simulink subsystem "Hall_Sensor_Reader"  (R2024b)
settings: Solver=VariableStepAuto  StartTime=0.0  StopTime=10.0  RelTol=1e-3
settings Model: Creator=luigi  LastModifiedBy=luigi

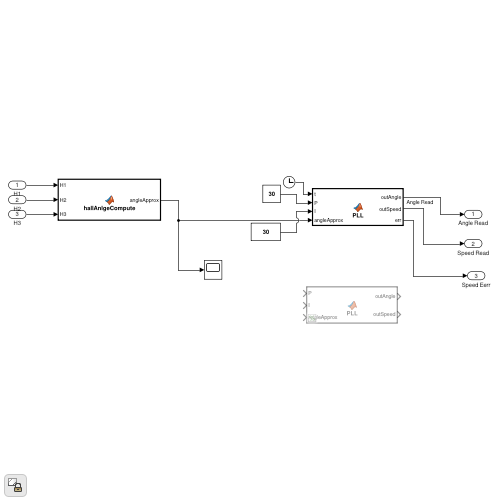
[thumbnail: Simulink's stored preview of the top-level diagram]
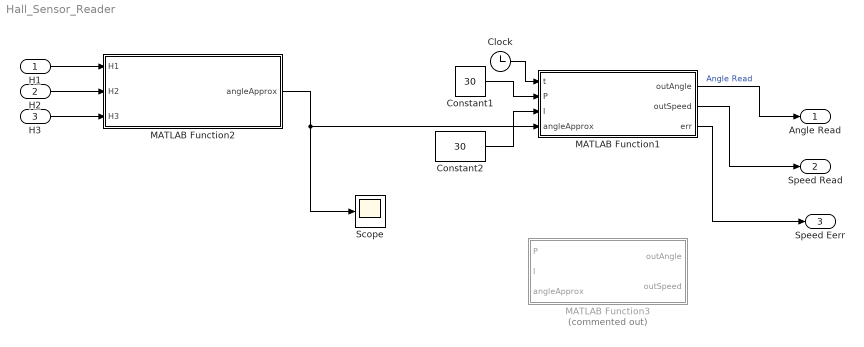
== system Hall_Sensor_Reader ==
  H1 : Inport
  H2 : Inport  Port=2
  H3 : Inport  Port=3
  Clock : Clock
  Constant1 : Constant  Value=30
  Constant2 : Constant  Value=30
  MATLAB Function1 : MATLAB Function  TreatAsAtomicUnit=on  SystemSampleTime=1e-3
  MATLAB Function2 : MATLAB Function  TreatAsAtomicUnit=on
  MATLAB Function3 : MATLAB Function  Commented=on  TreatAsAtomicUnit=on  SystemSampleTime=5e-4
  Scope : Scope
  Angle Read : Outport
  Speed Read : Outport  Port=2
  Speed Eerr : Outport  Port=3
  wires:
  H3/1 -> MATLAB Function2/3(H3)
  H1/1 -> MATLAB Function2/1(H1)
  Constant2/1 -> MATLAB Function1/3(I)
  Constant1/1 -> MATLAB Function1/2(P)
  H2/1 -> MATLAB Function2/2(H2)
  MATLAB Function2/1(angleApprox) -> MATLAB Function1/4(angleApprox), Scope/1
  MATLAB Function1/1(outAngle) -> Angle Read/1  "Angle Read"
  MATLAB Function1/2(outSpeed) -> Speed Read/1
  Clock/1 -> MATLAB Function1/1(t)
  MATLAB Function1/3(err) -> Speed Eerr/1

== matlab function Hall_Sensor_Reader/MATLAB Function1 ==
  data: t input; P input; outAngle output; I input; outSpeed output; angleApprox input; err output
function [outAngle, outSpeed, err] = PLL(t,P,I, angleApprox)
    Ts = 1e-3;
    persistent integral
    persistent fallEdge
    persistent oldAngle
    persistent oldTime
    persistent oldDuration
    persistent oldError
    persistent oldSpeed
    persistent outIntegral
    
    if isempty(oldDuration)
        oldDuration = 0;
    end
    if isempty(oldAngle)
        oldAngle = 0;
    end
    if isempty(oldSpeed)
        oldSpeed = 0;
    end
    if isempty(outIntegral)
        outIntegral = 0;
    end
    if isempty(fallEdge)
        fallEdge = 0;
    end
    if isempty(integral)
        integral = 0;
    end
    if isempty(oldError)
        oldError = 0;
    end
    if isempty(oldTime)
        oldTime = 0;
    end

    % Detect change in angle
    if oldAngle ~= angleApprox && fallEdge == 0


        if angleApprox == 0 && oldAngle ~= 0
            % If this is the last step of the sensor, do some tricks
            oldAngle = 2*pi;
            fallEdge = 1;
        else 
            oldAngle = angleApprox;
        end

        oldDuration = (t - oldTime);
        oldTime = t;
        oldError = (oldAngle) - (outIntegral);

        if oldError < 0 
            oldError = oldError * 100;
        end
           
    end

    if oldAngle == 2*pi && t - oldTime > (oldDuration/2)
        oldAngle = 0;
        fallEdge = 0;
    end

    if oldError < -pi
        oldError = oldError + 2*pi;
    elseif oldError > pi
        oldError = oldError - 2*pi;
    end
   


    % PLL's PID 
    u = oldError * P + integral * I * Ts;
    integral = integral + oldError;
    
    % Generate outputs
    outAngle = outIntegral;
    outSpeed = oldAngle;
    err = oldError;

    outIntegral = outIntegral + u * Ts;
    
    if outIntegral > 2*pi
        outIntegral = outIntegral - 2*pi;
    elseif outIntegral < -2*pi
        outIntegral = outIntegral + 2*pi;
    end

== matlab function Hall_Sensor_Reader/MATLAB Function2 ==
  settings: updateMethod=DISCRETE  sampleTime=1e-3
  data: H1 input uint8; H2 input uint8; H3 input uint8; angleApprox output
function angleApprox  = hallAnlgeCompute( H1, H2, H3)

    % HALL_OUT_LUT_60 = [1,0,1;1,0,0;1,1,0;0,1,0;0,1,1;0,0,1];
    
    hallReading = bitor(bitshift(H2, 1), bitshift(H3, 2));
    hallReading = bitor(hallReading, bitshift(H1, 0));

    angleApprox = 0;
    switch hallReading
        case 0b101
            angleApprox = 0;
        case 0b100
            angleApprox = pi/3;
        case 0b110
            angleApprox = 2*pi/3;
        case 0b010
            angleApprox = pi;
        case 0b011
            angleApprox = 4*pi/3;
        case 0b001
            angleApprox = 5*pi/3;
    end

end

== matlab function Hall_Sensor_Reader/MATLAB Function3 ==
  data: P input; outAngle output; I input; outSpeed output; angleApprox input
function [outAngle, outSpeed] = PLL(P,I, angleApprox)
    Ts = 5e-4;
    persistent integral
    persistent fallEdge
    persistent turnCount
    persistent outIntegral
    
    if isempty(turnCount)
        turnCount = 0;
    end

    if isempty(outIntegral)
        outIntegral = 0;
    end

    if isempty(fallEdge)
        fallEdge = 0;
    end

    if isempty(integral)
        integral = 0;
    end

    if angleApprox > 5 && fallEdge == 0
        fallEdge = -1;
        turnCount = turnCount + 1;
    end
    if fallEdge == -1 && angleApprox < 2
        fallEdge = 0;
    end

    if angleError > pi
        angleError = angleError - pi;
    elseif angleError < -pi
        angleError = angleError + pi;
    end
    % error = Ref - x;
    u = angleError * P + integral * I * Ts;

    integral = integral + angleError;
    
    outAngle = outIntegral;
    outSpeed = u;

    outIntegral = outIntegral + u * Ts;
    if outIntegral > 2*pi
        outIntegral = outIntegral - 2*pi;
    elseif outIntegral < -2*pi
        outIntegral = outIntegral + 2*pi;
    end
